simulink model "Electromagnetic_Torque_Calcu"  (R2020b)
settings: Solver=VariableStepAuto  StartTime=0.0  StopTime=10.0  RelTol=1e-3
model workspace (MAT data in the model file):
  J = Simulink.Parameter
  J.Value = 0.0002
  J.DataType = 'auto'
  J.Dimensions = [1 1]
  Ke = Simulink.Parameter
  Ke.Value = 0.1128
  Ke.DataType = 'auto'
  Ke.Dimensions = [1 1]
  L = Simulink.Parameter
  L.Value = 0.00272
  L.DataType = 'auto'
  L.Dimensions = [1 1]
  R = Simulink.Parameter
  R.Value = 0.7
  R.DataType = 'auto'
  R.Dimensions = [1 1]
  betaa = Simulink.Parameter
  betaa.Value = 2
  betaa.DataType = 'auto'
  betaa.Dimensions = [1 1]
  p = Simulink.Parameter
  p.Value = 4
  p.DataType = 'auto'
  p.Dimensions = [1 1]
  theta = Simulink.Parameter
  theta.DataType = 'auto'
  theta.Dimensions = [0 0]
settings Model: Creator=ASUS  LastModifiedBy=ASUS
settings DataIOCC: SaveOutput=off  SaveTime=off

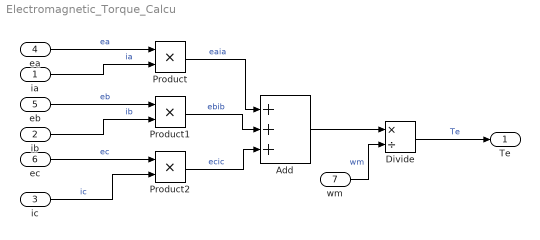
== system Electromagnetic_Torque_Calcu ==
  ia : Inport  OutDataTypeStr=double  PortDimensions=1  SampleTime=0
  ib : Inport  Port=2  OutDataTypeStr=double  PortDimensions=1  SampleTime=0
  ic : Inport  Port=3  OutDataTypeStr=double  PortDimensions=1  SampleTime=0
  ea : Inport  Port=4  OutDataTypeStr=double  PortDimensions=1  SampleTime=0
  eb : Inport  Port=5  OutDataTypeStr=double  PortDimensions=1  SampleTime=0
  ec : Inport  Port=6  OutDataTypeStr=double  PortDimensions=1  SampleTime=0
  wm : Inport  Port=7  OutDataTypeStr=double  PortDimensions=1  SampleTime=0
  Add : Sum  Inputs=+++
  Divide : Product  Inputs=*/
  Product : Product
  Product1 : Product
  Product2 : Product
  Te : Outport  OutDataTypeStr=double  PortDimensions=1  SampleTime=0
  wires:
  Divide/1 -> Te/1  "Te"
  Product/1 -> Add/1  "eaia"
  Product1/1 -> Add/2  "ebib"
  ic/1 -> Product2/2  "ic"
  ea/1 -> Product/1  "ea"
  Product2/1 -> Add/3  "ecic"
  Add/1 -> Divide/1
  ia/1 -> Product/2  "ia"
  wm/1 -> Divide/2  "wm"
  eb/1 -> Product1/1  "eb"
  ec/1 -> Product2/1  "ec"
  ib/1 -> Product1/2  "ib"
